simulink model "experiment"  (R2022a)
settings: Solver=VariableStepAuto  StartTime=0.0  StopTime=10  RelTol=1e-3
settings Model: Creator=Lenovo  LastModifiedBy=Lenovo

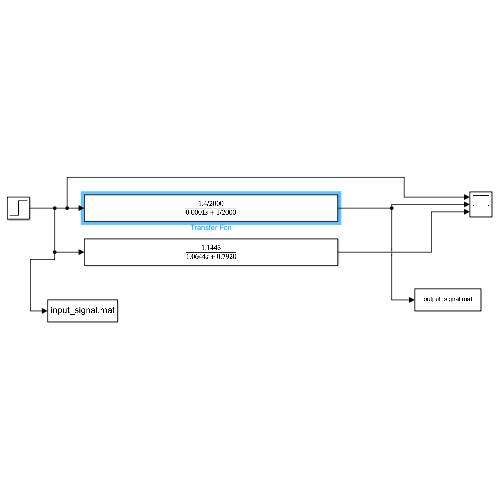
[thumbnail: Simulink's stored preview of the top-level diagram]
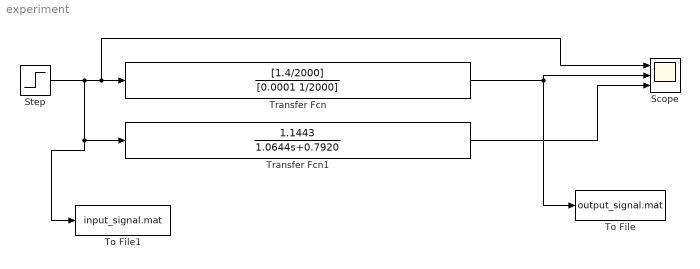
== system experiment ==
  Scope : Scope  NumInputPorts=3
  Step : Step  SampleTime=0
  To File : ToFile  Filename=output_signal.mat  MatrixName=out_signal  SampleTime=1
  To File1 : ToFile  Filename=input_signal.mat  MatrixName=in_signal  SampleTime=1
  Transfer Fcn : TransferFcn  Numerator=[1.4/2000]  Denominator=[0.0001 1/2000]
  Transfer Fcn1 : TransferFcn  Numerator=1.1443  Denominator=[1.0644 0.7920]
  wires:
  Step/1 -> Transfer Fcn1/1, To File1/1, Scope/1, Transfer Fcn/1
  Transfer Fcn/1 -> Scope/2, To File/1
  Transfer Fcn1/1 -> Scope/3
